simulink model "controller2"  (R2021b)
settings: Solver=ode45  StartTime=0.0  StopTime=15.0  RelTol=1e-3
libraries: cstblocks x2
settings Model: Creator=dabner  LastModifiedBy=dabner

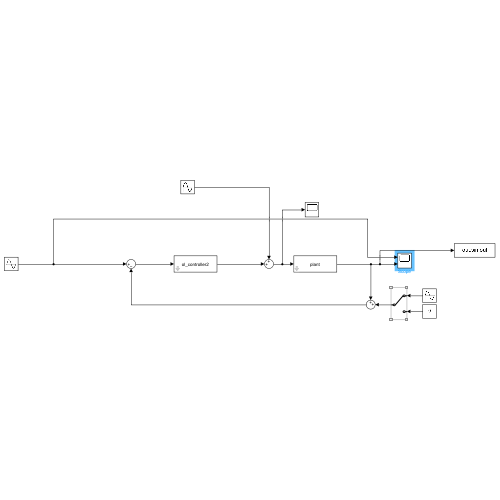
[thumbnail: Simulink's stored preview of the top-level diagram]
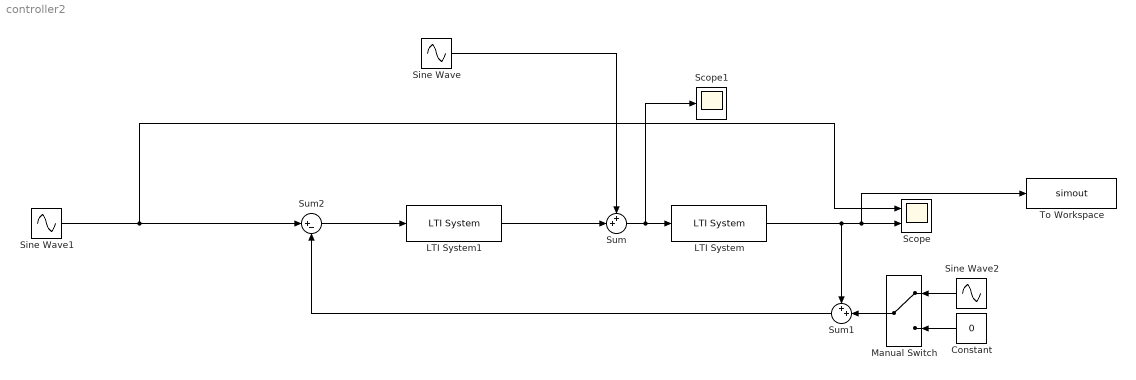
== system controller2 ==
  Constant : Constant  Value=0
  LTI System : cstblocks/LTI System  sys=plant  IC=[]
  LTI System1 : cstblocks/LTI System  sys=ol_controller2  IC=[]
  Manual Switch : ManualSwitch
  Scope : Scope  NumInputPorts=2
  Scope1 : Scope
  Sine Wave : Sin  Amplitude=.2  Frequency=2  SampleTime=0
  Sine Wave1 : Sin  Amplitude=3  Frequency=5  SampleTime=0
  Sine Wave2 : Sin  Frequency=20  SampleTime=0
  Sum : Sum  Inputs=++|
  Sum1 : Sum  Inputs=++|
  Sum2 : Sum  Inputs=|+-
  To Workspace : ToWorkspace  VariableName=simout  SampleTime=-1
      settings: Save2DSignal=2-D array (concatenate along first dimension)
  wires:
  LTI System/1 -> Sum1/1, To Workspace/1, Scope/2
  Sine Wave1/1 -> Sum2/1, Scope/1
  Sum/1 -> Scope1/1, LTI System/1
  Sum1/1 -> Sum2/2
  Sine Wave/1 -> Sum/1
  LTI System1/1 -> Sum/2
  Sum2/1 -> LTI System1/1
  Manual Switch/1 -> Sum1/2
  Sine Wave2/1 -> Manual Switch/1
  Constant/1 -> Manual Switch/2
